simulink model "propeller_power_train"  (R2023b)
settings: Solver=ode1be  StartTime=0.0  StopTime=simlength  FixedStep=tc  MaxStep=tc
values from neighbouring files (symbols this model uses):
  angle_error = angle_error_deg/180*pi    (= 0.13962634016)    [init_2023_10_06.m]
  CTRPIFF_CLIP_RELEASE = 0.01    [init_2023_10_06.m]
  dead_time = dead_time_INV    (= 4.2e-07)    [init_2023_10_06.m]
  dead_time_INV = 0.42e-6    (= 4.2e-07)    [init_2023_10_06.m]
  DThs_init = 0    [init_2023_10_06.m]
  emf_fb_p = 0.2    [init_2023_10_06.m]
  emf_fb_p_ccaller_1 = 0.2    [init_2023_10_06.m]
  emf_fb_p_ccaller_2 = 0.4    [init_2023_10_06.m]
  emf_p = emf_fb_p*4/10    (= 0.08)    [init_2023_10_06.m]
  emf_p_ccaller_1 = emf_fb_p_ccaller_1*4/10    (= 0.08)    [init_2023_10_06.m]
  emf_p_ccaller_2 = emf_fb_p_ccaller_2*4/10    (= 0.16)    [init_2023_10_06.m]
  fPWM_INV = 30e3    (= 30000)    [init_2023_10_06.m]
  g0_reference_flt = fcut_reference_flt * ts_inv * 2*pi    (= 0.000837758040957)    [init_2023_10_06.m]
  g1_reference_flt = 1 - g0_reference_flt    (= 0.999162241959)    [init_2023_10_06.m]
  id_ref_if_pu = iload_rms_ref*sqrt(2)/ibez    [init_2023_10_06.m]
  kg = K(1)    [init_2023_10_06.m]
  ki_id = 35    [init_2023_10_06.m]
  ki_iq = 35    [init_2023_10_06.m]
  kp_id = 0.15    [init_2023_10_06.m]
  kp_iq = 0.15    [init_2023_10_06.m]
  kw = K(2)    [init_2023_10_06.m]
  motorc_m_scale = 2/3*Vdc_bez/ubez    [init_2023_10_06.m]
  number_of_cells = 92    [init_2023_10_06.m]
  omega_flt_fcut = 4    [init_2023_10_06.m]
  omega_flt_g0 = omega_flt_fcut * ts_inv * 2*pi    (= 0.000837758040957)    [init_2023_10_06.m]
  omega_flt_g1 = 1 - omega_flt_g0    (= 0.999162241959)    [init_2023_10_06.m]
  omega_ref_if_pu = 300*2*pi/omega_bez    [init_2023_10_06.m]
  phase_compensation_omega = 0    [init_2023_10_06.m]
  pwm_out_lim = 1    [init_2023_10_06.m]
  Q = 10    [init_2023_10_06.m]
  q1Kalman = ts_inv^2    (= 1.11111111111e-09)    [init_2023_10_06.m]
  q2Kalman = ts_inv^1    (= 3.33333333333e-05)    [init_2023_10_06.m]
  q3Kalman = 0    [init_2023_10_06.m]
  rKalman = 1    [init_2023_10_06.m]
  Tambient = 1    [init_2023_10_06.m]
  tc = ts_inv/400    (= 8.33333333333e-08)    [init_2023_10_06.m]
  time_init = 0.025    [init_2023_10_06.m]
  torque_ref = 64/ibez*1.1    [init_2023_10_06.m]
  ts_inv = 1/fPWM_INV    (= 3.33333333333e-05)    [init_2023_10_06.m]
  tsample = ts_inv    (= 3.33333333333e-05)    [init_2023_10_06.m]
  Vdc_bez = 400    [init_2023_10_06.m]
undefined symbols (not defined in the file or in its folder): b, b_square, ibez, Jm, Ld_norm, Lq_norm, Ls_norm, magnitude, omega_bez, phi_bez, phi_m, phi_m_norm, R_RLload, Rload_eq, Rs_norm, tau_bez, weigth
libraries: fl_lib x90, nesl_utility x80, ee_lib x11, pmsm_uvw_with_harmonics_lib x2, lithium_ion_cell_lib x1, simulink x1, flexshaft_lib x1
(part 3 of 5)

== system propeller_power_train/driver control/current_ctrl/sample_hold_normalization ==
  iu : Inport
  iv : Inport  Port=2
  iw : Inport  Port=3
  Gain : Gain  Gain=1/ibez
  Gain1 : Gain  Gain=1/ibez
  Gain2 : Gain  Gain=1/ibez
  Gain3 : Gain  Commented=through  Gain=-1
  Gain4 : Gain  Commented=through  Gain=-1
  Gain5 : Gain  Commented=through  Gain=-1
  Unit Delay{,1..5} (6 alike) : UnitDelay  SampleTime=ts_inv  HasFrameUpgradeWarning=on
  Zero-Order Hold : ZeroOrderHold  SampleTime=ts_inv
  Zero-Order Hold1 : ZeroOrderHold  SampleTime=ts_inv
  Zero-Order Hold2 : ZeroOrderHold  SampleTime=ts_inv
  iu_pu : Outport
  iv_pu : Outport  Port=2
  iw_pu : Outport  Port=3
  wires:
  iv/1 -> Zero-Order Hold1/1
  iw/1 -> Zero-Order Hold2/1
  Zero-Order Hold/1 -> Unit Delay/1
  Zero-Order Hold2/1 -> Unit Delay4/1
  Unit Delay/1 -> Unit Delay2/1
  Zero-Order Hold1/1 -> Unit Delay1/1
  Unit Delay1/1 -> Unit Delay3/1
  Unit Delay4/1 -> Unit Delay5/1
  iu/1 -> Zero-Order Hold/1
  Gain/1 -> Gain3/1
  Gain1/1 -> Gain4/1
  Gain2/1 -> Gain5/1
  Gain3/1 -> iu_pu/1
  Gain4/1 -> iv_pu/1
  Gain5/1 -> iw_pu/1
  Unit Delay2/1 -> Gain/1
  Unit Delay3/1 -> Gain1/1
  Unit Delay5/1 -> Gain2/1

== system propeller_power_train/driver control/current_ctrl/vector_current_ctrl ==
  iq_ref : Inport
  id_ref : Inport  Port=2
  MTPA : Subsystem
      settings: PortSchema="{\"entries\":[{\"content\":{\"sides\":[{\"content\":{\"connectorIds\":[\"In1\"]},\"type\":\"ConnectorPlacement.EquallySpacedRectSide\",\"uuid\":\"b7b50820-32cf-4b06-b710-c36db40508fb\"},{\"content\":{\"connectorIds\":[\"Out1\"],\"side\":\"RIGHT\"},\"type\":\"ConnectorPlacement.EquallySpacedRectSide\",\"uuid\":\"9680176d-6365-4ae4-8330-83815ae14f93\"},{\"content\":{\"connectorIds\":[\"In2\"],\"side\":\"TOP\"},\"type\":\"ConnectorPlacement.EquallySpacedRectSide\",\"uuid\":\"503d8594-1c43-4fac-b8a6-77f5afdeeec1\"}]},\"type\":\"ConnectorPlacement.EquallySpacedConnector\",\"uuid\":\"c97785bf-1f92-4066-ba86-64cef6027105\"}],\"packageUris\":[\"http://schema.mathworks.com/mf0/Connector/R2020b\"],\"version\":\"1.0\"}"
  Variant Source : VariantSource  ShowConditionOnBlock=on
  Variant Source1 : VariantSource  ShowConditionOnBlock=on
  dq_vector_pi : Subsystem
  dq_vector_pi_ccaller : Subsystem
  id_ref_pu/id_pu : Scope  NumInputPorts=2
  iq_ref_pu/iq_pu : Scope  NumInputPorts=2
  ud : Outport
  uq : Outport  Port=2
  tag scope: id_ref_inverter_pu=global, iq_ref_inverter_pu=global, ud_inverter_pu=global, uq_inverter_pu=global
  wires:
  [iq_inverter_pu] -> dq_vector_pi/3(iq), iq_ref_pu/iq_pu/2, dq_vector_pi_ccaller/3(iq)  "iq_inverter_pu"
  [id_inverter_pu] -> dq_vector_pi/1(id), dq_vector_pi_ccaller/1(id), id_ref_pu/id_pu/2  "id_inverter_pu"
  iq_ref/1 -> MTPA/1(iq_ref), dq_vector_pi/4(iq_ref), [iq_ref_inverter_pu], iq_ref_pu/iq_pu/1, dq_vector_pi_ccaller/4(iq_ref)  "iq_ref"
  MTPA/1(id_ref) -> dq_vector_pi/2(id_ref), dq_vector_pi_ccaller/2(id_ref), [id_ref_inverter_pu], id_ref_pu/id_pu/1  "id_ref"
  id_ref/1 -> MTPA/2(id_ref_ext)
  Variant Source/1 -> [ud_inverter_pu], ud/1
  dq_vector_pi_ccaller/1(ud_ctrl_out) -> Variant Source/1
  dq_vector_pi_ccaller/2(uq_ctrl_out) -> Variant Source1/1
  Variant Source1/1 -> [uq_inverter_pu], uq/1
  dq_vector_pi/1(ctrl_d_u) -> Variant Source/2
  dq_vector_pi/2(ctrl_q_u) -> Variant Source1/2

== system propeller_power_train/driver control/torque_reference_generator/reference_d_flt ==
  input : Inport
  Gain3 : Gain  Gain=g1_reference_flt
  Gain6 : Gain  Gain=g0_reference_flt
  Sum : Sum  Inputs=|++
  Unit Delay1 : UnitDelay  SampleTime=ts_inv  HasFrameUpgradeWarning=on
  output : Outport  VectorParamsAs1DForOutWhenUnconnected=off
  wires:
  Gain6/1 -> Sum/1
  input/1 -> Gain6/1
  Unit Delay1/1 -> Gain3/1
  Gain3/1 -> Sum/2
  Sum/1 -> Unit Delay1/1, output/1

== system propeller_power_train/driver control/torque_reference_generator/reference_q_flt ==
  input : Inport
  Gain3 : Gain  Gain=g1_reference_flt
  Gain6 : Gain  Gain=g0_reference_flt
  Sum : Sum  Inputs=|++
  Unit Delay1 : UnitDelay  SampleTime=ts_inv  HasFrameUpgradeWarning=on
  output : Outport  VectorParamsAs1DForOutWhenUnconnected=off
  wires:
  Sum/1 -> output/1, Unit Delay1/1
  Gain3/1 -> Sum/2
  Unit Delay1/1 -> Gain3/1
  input/1 -> Gain6/1
  Gain6/1 -> Sum/1

== system propeller_power_train/inverter/Gyro based inverter/gyro1 ==
  m : Inport
  Controlled Current Source : fl_lib/Electrical/Electrical Sources/Controlled Current Source
  Controlled Voltage Source : fl_lib/Electrical/Electrical Sources/Controlled Voltage Source
  Current Sensor : fl_lib/Electrical/Electrical Sensors/Current Sensor
  PS Product : fl_lib/Physical Signals/Functions/PS Product
  PS Product1 : fl_lib/Physical Signals/Functions/PS Product
  Simulink-PS Converter : nesl_utility/Simulink-PS Converter  PhysicalDomain=network_engine_domain  SubClassName=ps_input  LeftPortType=input  RightPortType=output  PseudoPeriodic=off  Frequencies=[]  NoiseDistribution=none  NoiseParameters=[]  Unit=1  AffineConversion=on  FilteringAndDerivatives=provide  SimscapeFilterOrder=1  InputFilterTimeConstant=0.001  UdotUserProvided=0
  Voltage Sensor : fl_lib/Electrical/Electrical Sensors/Voltage Sensor
  uin+ : PMIOPort  Side=Left
  uin- : PMIOPort  Port=2  Side=Left
  uout+ : PMIOPort  Port=3  Side=Right
  uout- : PMIOPort  Port=4  Side=Right
  wires:
  m/1 -> Simulink-PS Converter/1
  connections:
  Voltage Sensor/RConn2 -- Controlled Current Source/LConn1 -- uin-/RConn1
  Voltage Sensor/LConn1 -- Controlled Current Source/RConn2 -- uin+/RConn1
  Controlled Voltage Source/LConn1 -- Current Sensor/LConn1
  Controlled Voltage Source/RConn2 -- uout-/RConn1
  Current Sensor/RConn2 -- uout+/RConn1
  Simulink-PS Converter/RConn1 -- PS Product/LConn1 -- PS Product1/LConn2
  Voltage Sensor/RConn1 -- PS Product/LConn2
  PS Product1/RConn1 -- Controlled Current Source/RConn1
  PS Product/RConn1 -- Controlled Voltage Source/RConn1
  Current Sensor/RConn1 -- PS Product1/LConn1

== system propeller_power_train/inverter/Gyro based inverter/gyro2 ==
  m : Inport
  Controlled Current Source : fl_lib/Electrical/Electrical Sources/Controlled Current Source
  Controlled Voltage Source : fl_lib/Electrical/Electrical Sources/Controlled Voltage Source
  Current Sensor : fl_lib/Electrical/Electrical Sensors/Current Sensor
  PS Product : fl_lib/Physical Signals/Functions/PS Product
  PS Product1 : fl_lib/Physical Signals/Functions/PS Product
  Simulink-PS Converter : nesl_utility/Simulink-PS Converter  PhysicalDomain=network_engine_domain  SubClassName=ps_input  LeftPortType=input  RightPortType=output  PseudoPeriodic=off  Frequencies=[]  NoiseDistribution=none  NoiseParameters=[]  Unit=1  AffineConversion=on  FilteringAndDerivatives=provide  SimscapeFilterOrder=1  InputFilterTimeConstant=0.001  UdotUserProvided=0
  Voltage Sensor : fl_lib/Electrical/Electrical Sensors/Voltage Sensor
  uin+ : PMIOPort  Side=Left
  uin- : PMIOPort  Port=2  Side=Left
  uout+ : PMIOPort  Port=3  Side=Right
  uout- : PMIOPort  Port=4  Side=Right
  wires:
  m/1 -> Simulink-PS Converter/1
  connections:
  Current Sensor/RConn1 -- PS Product1/LConn1
  PS Product/RConn1 -- Controlled Voltage Source/RConn1
  PS Product1/RConn1 -- Controlled Current Source/RConn1
  Voltage Sensor/RConn1 -- PS Product/LConn2
  PS Product1/LConn2 -- PS Product/LConn1 -- Simulink-PS Converter/RConn1
  Current Sensor/RConn2 -- uout+/RConn1
  Controlled Voltage Source/RConn2 -- uout-/RConn1
  Controlled Voltage Source/LConn1 -- Current Sensor/LConn1
  uin+/RConn1 -- Controlled Current Source/RConn2 -- Voltage Sensor/LConn1
  uin-/RConn1 -- Controlled Current Source/LConn1 -- Voltage Sensor/RConn2

== system propeller_power_train/inverter/Gyro based inverter/gyro3 ==
  m : Inport
  Controlled Current Source : fl_lib/Electrical/Electrical Sources/Controlled Current Source
  Controlled Voltage Source : fl_lib/Electrical/Electrical Sources/Controlled Voltage Source
  Current Sensor : fl_lib/Electrical/Electrical Sensors/Current Sensor
  PS Product : fl_lib/Physical Signals/Functions/PS Product
  PS Product1 : fl_lib/Physical Signals/Functions/PS Product
  Simulink-PS Converter : nesl_utility/Simulink-PS Converter  PhysicalDomain=network_engine_domain  SubClassName=ps_input  LeftPortType=input  RightPortType=output  PseudoPeriodic=off  Frequencies=[]  NoiseDistribution=none  NoiseParameters=[]  Unit=1  AffineConversion=on  FilteringAndDerivatives=provide  SimscapeFilterOrder=1  InputFilterTimeConstant=0.001  UdotUserProvided=0
  Voltage Sensor : fl_lib/Electrical/Electrical Sensors/Voltage Sensor
  uin+ : PMIOPort  Side=Left
  uin- : PMIOPort  Port=2  Side=Left
  uout+ : PMIOPort  Port=3  Side=Right
  uout- : PMIOPort  Port=4  Side=Right
  wires:
  m/1 -> Simulink-PS Converter/1
  connections:
  Voltage Sensor/RConn2 -- Controlled Current Source/LConn1 -- uin-/RConn1
  Voltage Sensor/LConn1 -- Controlled Current Source/RConn2 -- uin+/RConn1
  Controlled Voltage Source/LConn1 -- Current Sensor/LConn1
  Controlled Voltage Source/RConn2 -- uout-/RConn1
  Current Sensor/RConn2 -- uout+/RConn1
  Simulink-PS Converter/RConn1 -- PS Product/LConn1 -- PS Product1/LConn2
  Voltage Sensor/RConn1 -- PS Product/LConn2
  PS Product1/RConn1 -- Controlled Current Source/RConn1
  PS Product/RConn1 -- Controlled Voltage Source/RConn1
  Current Sensor/RConn1 -- PS Product1/LConn1

== system propeller_power_train/inverter/MOS based inverter/inverter ==
  inverter_mosfet_leg_thermal : Subsystem
  inverter_without_mosfet_leg_thermal : Subsystem  Commented=on
  udc(+) : PMIOPort  Side=Left
  udc(-) : PMIOPort  Port=2  Side=Left
  u : PMIOPort  Port=3  Side=Right
  v : PMIOPort  Port=4  Side=Right
  w : PMIOPort  Port=5  Side=Right
  connections:
  udc(+)/RConn1 -- inverter_without_mosfet_leg_thermal/LConn1 -- inverter_mosfet_leg_thermal/LConn1
  inverter_mosfet_leg_thermal/RConn1 -- inverter_without_mosfet_leg_thermal/RConn1 -- u/RConn1
  inverter_mosfet_leg_thermal/RConn2 -- inverter_without_mosfet_leg_thermal/RConn2 -- v/RConn1
  w/RConn1 -- inverter_without_mosfet_leg_thermal/RConn3 -- inverter_mosfet_leg_thermal/RConn3
  udc(-)/RConn1 -- inverter_without_mosfet_leg_thermal/LConn2 -- inverter_mosfet_leg_thermal/LConn2

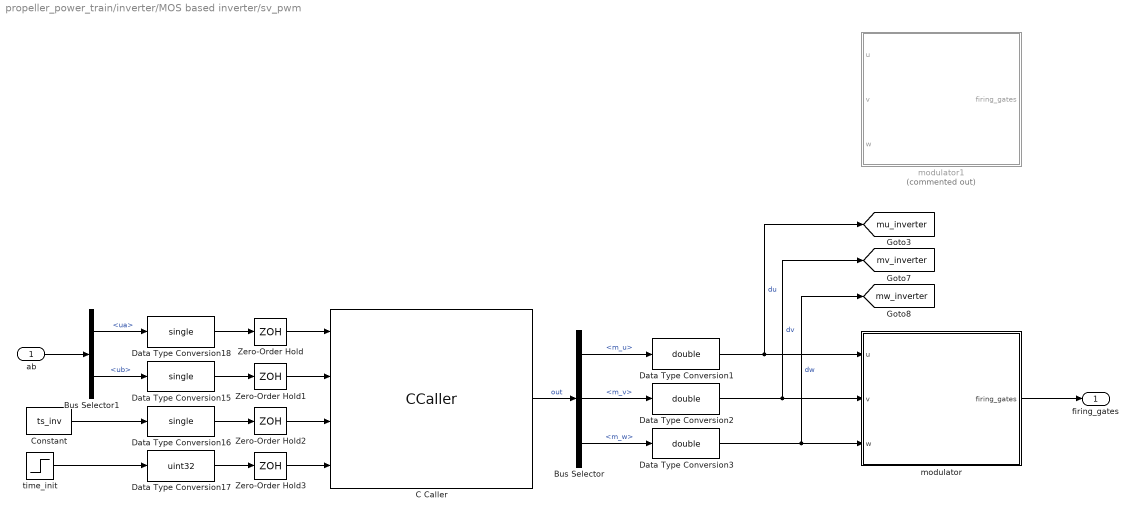
== system propeller_power_train/inverter/MOS based inverter/sv_pwm ==
  ab : Inport
  Bus Selector : BusSelector  OutputSignals=m_u,m_v,m_w
  Bus Selector1 : BusSelector  OutputSignals=ua,ub
  C Caller : CCaller  FunctionName=sv_pwm_process_simulink  PortSpecificationStruct="%)30     .    N @   8    (     @         %    \"     4    !     0         %  0 \"0    $    _    07)G3F%M90  4&]R=$YA;64 4V-O<&4     26YD97@     5'EP90      4VEZ90      27-';&]B86P   X    P    !@    @    $          4    (     0    ,    !         !   P!O=70 #@   #     &    \"     0         !0    @    !     P    $         $  # &]U=  .    .     8    (    !          %    \"     $    &     0         0   ...(+2630 chars)"  SampleTime=ts_inv
  Constant : Constant  Value=ts_inv
  Data Type Conversion1 : DataTypeConversion  OutDataTypeStr=double  SaturateOnIntegerOverflow=off  RndMeth=Floor
  Data Type Conversion15 : DataTypeConversion  OutDataTypeStr=single  SaturateOnIntegerOverflow=off  RndMeth=Floor
  Data Type Conversion16 : DataTypeConversion  OutDataTypeStr=single  SaturateOnIntegerOverflow=off  RndMeth=Floor
  Data Type Conversion17 : DataTypeConversion  OutDataTypeStr=uint32  SaturateOnIntegerOverflow=off  RndMeth=Floor
  Data Type Conversion18 : DataTypeConversion  OutDataTypeStr=single  SaturateOnIntegerOverflow=off  RndMeth=Floor
  Data Type Conversion2 : DataTypeConversion  OutDataTypeStr=double  SaturateOnIntegerOverflow=off  RndMeth=Floor
  Data Type Conversion3 : DataTypeConversion  OutDataTypeStr=double  SaturateOnIntegerOverflow=off  RndMeth=Floor
  Zero-Order Hold{,1..3} (4 alike) : ZeroOrderHold  SampleTime=ts_inv
  modulator : Subsystem
  modulator1 : Subsystem  Commented=on
  time_init : Step  Time=time_init  SampleTime=0
  firing_gates : Outport
  tag scope: mu_inverter=global, mv_inverter=global, mw_inverter=global
  wires:
  Data Type Conversion1/1 -> [mu_inverter], modulator/1(u)  "du"
  Zero-Order Hold/1 -> C Caller/1
  Zero-Order Hold2/1 -> C Caller/3
  Constant/1 -> Data Type Conversion16/1
  Bus Selector/1 -> Data Type Conversion1/1  "<m_u>"
  Data Type Conversion18/1 -> Zero-Order Hold/1
  Bus Selector/3 -> Data Type Conversion3/1  "<m_w>"
  Data Type Conversion2/1 -> [mv_inverter], modulator/2(v)  "dv"
  Data Type Conversion16/1 -> Zero-Order Hold2/1
  Zero-Order Hold1/1 -> C Caller/2
  Data Type Conversion17/1 -> Zero-Order Hold3/1
  Zero-Order Hold3/1 -> C Caller/4
  Data Type Conversion15/1 -> Zero-Order Hold1/1
  C Caller/1 -> Bus Selector/1  "out"
  Bus Selector/2 -> Data Type Conversion2/1  "<m_v>"
  Data Type Conversion3/1 -> [mw_inverter], modulator/3(w)  "dw"
  modulator/1(firing_gates) -> firing_gates/1
  ab/1 -> Bus Selector1/1
  Bus Selector1/1 -> Data Type Conversion18/1  "<ua>"
  Bus Selector1/2 -> Data Type Conversion15/1  "<ub>"
  time_init/1 -> Data Type Conversion17/1

== system propeller_power_train/inverter/MOS based inverter/threePhsModulator ==
  uab_pu : Inport
  Bus Creator1 : BusCreator  Inputs=2
  Bus Creator2 : BusCreator  Inputs=2
  Bus Creator3 : BusCreator  Inputs=3
  Bus Creator4 : BusCreator  Inputs=2
  Demux1 : Demux  Outputs=2
  Gain6 : Gain  Gain=1/sqrt(3)*2
  Gain7 : Gain  Gain=1/sqrt(3)*2
  Gain8 : Gain  Gain=1/sqrt(3)*2
  PWM generator 1 : Subsystem  mask{f=fPWM_INV, ph=0, m_up=1, m_low=-1, dead_time=dead_time, gate_voltage=15}
      mask prompts: f "Frequency"; ph "Phase"; m_up "Max Input Modulation Value"; m_low "Min Input Modulation Value"; dead_time "Dead Time"; gate_voltage "Gate Voltage"
  PWM generator 2 : Subsystem  mask{f=fPWM_INV, ph=0, m_up=1, m_low=-1, dead_time=dead_time, gate_voltage=15}
      mask prompts: f "Frequency"; ph "Phase"; m_up "Max Input Modulation Value"; m_low "Min Input Modulation Value"; dead_time "Dead Time"; gate_voltage "Gate Voltage"
  PWM generator 3 : Subsystem  mask{f=fPWM_INV, ph=0, m_up=1, m_low=-1, dead_time=dead_time, gate_voltage=15}
      mask prompts: f "Frequency"; ph "Phase"; m_up "Max Input Modulation Value"; m_low "Min Input Modulation Value"; dead_time "Dead Time"; gate_voltage "Gate Voltage"
  Sum : Sum  Inputs=|+-
  Sum1 : Sum  Inputs=|+-
  Sum2 : Sum  Inputs=|+-
  Third harmonic injecting : Subsystem
  du/dv/dw : Scope  NumInputPorts=3
  uvw2alphabeta1 : MATLAB Function  TreatAsAtomicUnit=on  SystemSampleTime=ts_inv
  mout : Outport
  wires:
  uab_pu/1 -> Demux1/1
  Demux1/1 -> uvw2alphabeta1/1(alpha)
  Demux1/2 -> uvw2alphabeta1/2(beta)
  Third harmonic injecting/1(thind_H) -> Sum1/2, Sum/2, Sum2/2
  uvw2alphabeta1/1(u) -> Third harmonic injecting/1(m1), Sum/1  "ur"
  uvw2alphabeta1/2(v) -> Third harmonic injecting/2(m2), Sum1/1  "vr"
  uvw2alphabeta1/3(w) -> Sum2/1, Third harmonic injecting/3(m3)  "wr"
  Sum/1 -> Gain6/1
  Bus Creator3/1 -> mout/1
  PWM generator 1/1(m1) -> Bus Creator1/1  "gate_command_1"
  PWM generator 1/2(m2) -> Bus Creator1/2  "gate_command_2"
  Bus Creator1/1 -> Bus Creator3/1  "legA"
  PWM generator 2/2(m2) -> Bus Creator2/2  "gate_command_4"
  PWM generator 2/1(m1) -> Bus Creator2/1  "gate_command_3"
  PWM generator 3/1(m1) -> Bus Creator4/1  "gate_command_5"
  PWM generator 3/2(m2) -> Bus Creator4/2  "gate_command_6"
  Bus Creator2/1 -> Bus Creator3/2  "legB"
  Bus Creator4/1 -> Bus Creator3/3  "legC"
  Sum1/1 -> Gain7/1
  Sum2/1 -> Gain8/1
  Gain6/1 -> du/dv/dw/1, PWM generator 1/1(m_index)  "mu"
  Gain8/1 -> du/dv/dw/3, PWM generator 3/1(m_index)  "mw"
  Gain7/1 -> PWM generator 2/1(m_index), du/dv/dw/2  "mv"

== system propeller_power_train/battery_system/battery_system/LithiumIonBattery/SOC_estimator ==
  Kalman_observer : Subsystem
  SOC*/SOC : Scope  Commented=on  NumInputPorts=2
  Selector1 : Selector  InputPortWidth=3  IndexOptions=Index vector (dialog)  Indices=3  OutputSizes=1
  h_hat/h : Scope  Commented=on  NumInputPorts=2
  i_out/v_out : Scope  Commented=on  NumInputPorts=2
  soc/iout : Scope  Commented=on  NumInputPorts=2
  wires:
  Kalman_observer/2(SOC) -> SOC*/SOC/2
  Kalman_observer/1(x(k+1|k)) -> Selector1/1
  [im] -> i_out/v_out/1  "im+noise"
  [h] -> h_hat/h/2
  [SOC] -> soc/iout/1, SOC*/SOC/1
  Selector1/1 -> h_hat/h/1  "h_hat(z)"
  [vout] -> Kalman_observer/1(vout(k)), i_out/v_out/2
  [icell] -> soc/iout/2

== system propeller_power_train/battery_system/battery_system/LithiumIonBattery/lithium ion cell analytical ocv ==
  Current Sensor : fl_lib/Electrical/Electrical Sensors/Current Sensor
  Electrical Reference : fl_lib/Electrical/Electrical Elements/Electrical Reference
  PS Constant : fl_lib/Physical Signals/Sources/PS Constant  constant=298.15 K
  PS-Simulink Converter{,1..4} (5 alike) : nesl_utility/PS-Simulink Converter  PhysicalDomain=network_engine_domain  SubClassName=ps_output  LeftPortType=input  RightPortType=output  PseudoPeriodic=off  Frequencies=[]  VectorFormat=1-D array  Unit=inherit  AffineConversion=off
  Voltage Sensor : fl_lib/Electrical/Electrical Sensors/Voltage Sensor
  lithium-ion battery with analytical OCV : lithium_ion_cell_lib/lithium-ion Cell with analytical OCV  Qcell=Q hr*A  N=number_of_cells  E_1=E1 V  E0=E0 V  E1=E1 V  E2=E2 V  E3=E3 V  Elog=Elog V  R0=R0 Ohm  R1=R1 Ohm  C1=C1 F  M=M V  alpha=alpha  u_specify=off  u_priority=High  u=Vdc V  u_nominal_specify=off  u_nominal_unit=V  u_nominal_value=1  u_ocv_specify=off  u_ocv_priority=High  u_ocv=Vdc V  u_ocv_nominal_specify=off  u_ocv_nominal_unit=V  u_ocv_nominal_value=1  icell_specify=off  icell_priority=None  icell=0 A  icell_nominal_specify=off  icell_nominal_unit=A  icell_nominal_value=1  i_r1_specify=off  i_r1_priority=None  i_r1=0 A  i_r1_nominal_specify=off  i_r1_nominal_unit=A  i_r1_nominal_value=1  z_specify=on  z_priority=High  z=soc_init  z_nominal_specify=off  z_nominal_unit=1  z_nominal_value=1  h_specify=off  h_priority=High  h=0  h_nominal_specify=off  h_nominal_unit=1  h_nominal_value=1
      settings: InternalSimscapePortConfiguration="{\"Bottom\":[],\"Left\":[{\"id\":\"T\",\"label\":\"T\",\"type\":\"input\"}],\"Right\":[{\"id\":\"u_p\",\"label\":\"u+\",\"type\":\"foundation.electrical.electrical\"},{\"id\":\"u_n\",\"label\":\"u-\",\"type\":\"foundation.electrical.electrical\"},{\"id\":\"z_out\",\"label\":\"SOC\",\"type\":\"output\"},{\"id\":\"i_r1_out\",\"label\":\"i_r1\",\"type\":\"output\"},{\"id\":\"h_out\",\"label\":\"hysteresis\",\"type\":\"output\"}],\"Top\":[]}"
  white_noise : Subsystem
  U+ : PMIOPort  Side=Right
  U- : PMIOPort  Port=2  Side=Right
  tag scope: SOC=global, h=global, icell=global, im=global, vout=global
  wires:
  PS-Simulink Converter/1 -> [vout]  "vout(k)"
  PS-Simulink Converter1/1 -> white_noise/1(in)  "i(k)"
  white_noise/1(out) -> [im]
  PS-Simulink Converter4/1 -> [h]  "h(t)"
  PS-Simulink Converter2/1 -> [icell]  "icell"
  PS-Simulink Converter3/1 -> [SOC]  "SOC*"
  connections:
  lithium-ion battery with analytical OCV/LConn1 -- PS Constant/RConn1
  PS-Simulink Converter/LConn1 -- Voltage Sensor/RConn1
  Current Sensor/RConn2 -- Voltage Sensor/LConn1 -- U+/RConn1
  Electrical Reference/LConn1 -- Voltage Sensor/RConn2 -- U-/RConn1 -- lithium-ion battery with analytical OCV/RConn2
  Current Sensor/RConn1 -- PS-Simulink Converter1/LConn1
  lithium-ion battery with analytical OCV/RConn1 -- Current Sensor/LConn1
  lithium-ion battery with analytical OCV/RConn3 -- PS-Simulink Converter3/LConn1
  lithium-ion battery with analytical OCV/RConn4 -- PS-Simulink Converter2/LConn1
  lithium-ion battery with analytical OCV/RConn5 -- PS-Simulink Converter4/LConn1

== system propeller_power_train/driver control/bemf_observer/bemf_observer/double_integrator_observer ==
  theta : Inport
  Gain : Gain  Gain=kw
  Gain1 : Gain  Gain=kg
  Gain2 : Gain  Gain=omega_bez
  Gain3 : Gain  Gain=1/omega_bez
  Gain5 : Gain  Gain=ts_inv
  Sum : Sum  Inputs=-+|
  Sum1 : Sum  Inputs=|++
  Sum2 : Sum  Inputs=|++
  Sum8 : Sum  Inputs=++|
  Unit Delay1 : UnitDelay  SampleTime=ts_inv  HasFrameUpgradeWarning=on
  Unit Delay2 : UnitDelay  SampleTime=ts_inv  HasFrameUpgradeWarning=on
  bounder1 : MATLAB Function  TreatAsAtomicUnit=on  SystemSampleTime=ts_inv
  bounder2 : MATLAB Function  TreatAsAtomicUnit=on  SystemSampleTime=ts_inv
  omega_pu_hat : Outport  VectorParamsAs1DForOutWhenUnconnected=off
  theta_hat : Outport  Port=2  VectorParamsAs1DForOutWhenUnconnected=off
  wires:
  Gain1/1 -> Sum2/1
  theta/1 -> Sum/2  "theta_bemf"
  Sum8/1 -> bounder2/1(u)
  Sum1/1 -> Unit Delay2/1
  Gain/1 -> Gain3/1
  Unit Delay2/1 -> omega_pu_hat/1, Sum1/2, Gain5/1
  Sum2/1 -> Sum8/2
  bounder2/1(y) -> Unit Delay1/1
  bounder1/1(y) -> Gain/1, Gain1/1
  Gain2/1 -> Sum8/1
  Gain3/1 -> Sum1/1
  Gain5/1 -> Gain2/1
  Sum/1 -> bounder1/1(u)
  Unit Delay1/1 -> Sum2/2, theta_hat/1, Sum/1  "theta_hat"

== system propeller_power_train/driver control/bemf_observer/bemf_observer/omega_hat_flt ==
  omega_hat : Inport
  Gain3 : Gain  Gain=omega_flt_g1
  Gain6 : Gain  Gain=omega_flt_g0
  Sum : Sum  Inputs=|++
  Unit Delay1 : UnitDelay  SampleTime=ts_inv  HasFrameUpgradeWarning=on
  omega_hat_flt : Outport  VectorParamsAs1DForOutWhenUnconnected=off
  wires:
  Gain6/1 -> Sum/1
  omega_hat/1 -> Gain6/1
  Unit Delay1/1 -> Gain3/1
  Gain3/1 -> Sum/2
  Sum/1 -> Unit Delay1/1, omega_hat_flt/1

== system propeller_power_train/driver control/bemf_observer/bemf_observer/psi_alpha_hat ==
  ualpha : Inport
  ialpha : Inport  Port=2
  Gain1 : Gain  Gain=Rs_norm
  Gain2 : Gain  Gain=emf_fb_p
  Gain3 : Gain  Gain=emf_p
  Gain4 : Gain  Gain=omega_bez
  Gain5 : Gain  Gain=Ls_norm
  Gain6 : Gain  Gain=motorc_m_scale
  Gain7 : Gain  Gain=ts_inv
  Product : Product  RndMeth=Zero
  Sum : Sum  Inputs=|+-
  Sum1 : Sum  Inputs=|+-
  Sum2 : Sum  Inputs=++-  SaturateOnIntegerOverflow=on
  Sum3 : Sum  Inputs=|++
  Sum4 : Sum  Inputs=+-  SaturateOnIntegerOverflow=on
  Unit Delay1 : UnitDelay  SampleTime=ts_inv  HasFrameUpgradeWarning=on
  Unit Delay2 : UnitDelay  SampleTime=ts_inv  HasFrameUpgradeWarning=on
  Unit Delay3 : UnitDelay  SampleTime=ts_inv  HasFrameUpgradeWarning=on
  psi_s_alpha_hat : Outport  VectorParamsAs1DForOutWhenUnconnected=off
  psi_r_alpha_hat : Outport  Port=2  VectorParamsAs1DForOutWhenUnconnected=off
  wires:
  [psi_r_m_alpha] -> Sum1/1
  [psi_r_alpha_hat] -> Sum1/2
  Gain4/1 -> Gain7/1
  Sum2/1 -> Gain4/1
  Gain3/1 -> Sum2/3
  ialpha/1 -> Gain5/1, Gain1/1
  Gain1/1 -> Sum/2
  Sum/1 -> Sum2/2
  ualpha/1 -> Product/1
  Unit Delay1/1 -> Sum4/1, psi_s_alpha_hat/1, Gain3/1, Sum3/2
  Sum3/1 -> Unit Delay1/1  "psi_s_alpha_hat_hat"
  Sum1/1 -> Gain2/1
  Gain2/1 -> Sum2/1
  [vdc_pu] -> Product/2
  Gain7/1 -> Sum3/1
  Product/1 -> Gain6/1
  Gain6/1 -> Sum/1
  Gain5/1 -> Unit Delay2/1
  Sum4/1 -> Unit Delay3/1
  Unit Delay2/1 -> Sum4/2
  Unit Delay3/1 -> psi_r_alpha_hat/1

== system propeller_power_train/driver control/bemf_observer/bemf_observer/psi_beta_hat ==
  ubeta : Inport
  ibeta : Inport  Port=2
  Gain1 : Gain  Gain=Rs_norm
  Gain2 : Gain  Gain=emf_fb_p
  Gain3 : Gain  Gain=emf_p
  Gain4 : Gain  Gain=omega_bez
  Gain5 : Gain  Gain=Ls_norm
  Gain6 : Gain  Gain=motorc_m_scale
  Gain7 : Gain  Gain=ts_inv
  Product : Product  RndMeth=Zero
  Sum : Sum  Inputs=|+-
  Sum1 : Sum  Inputs=|+-
  Sum2 : Sum  Inputs=++-  SaturateOnIntegerOverflow=on
  Sum3 : Sum  Inputs=|++
  Sum4 : Sum  Inputs=+-  SaturateOnIntegerOverflow=on
  Unit Delay1 : UnitDelay  SampleTime=ts_inv  HasFrameUpgradeWarning=on
  Unit Delay2 : UnitDelay  SampleTime=ts_inv  HasFrameUpgradeWarning=on
  Unit Delay3 : UnitDelay  SampleTime=ts_inv  HasFrameUpgradeWarning=on
  psi_s_beta_hat : Outport  VectorParamsAs1DForOutWhenUnconnected=off
  psi_r_beta_hat : Outport  Port=2  VectorParamsAs1DForOutWhenUnconnected=off
  wires:
  Sum/1 -> Sum2/2
  Gain1/1 -> Sum/2
  ibeta/1 -> Gain5/1, Gain1/1
  Gain3/1 -> Sum2/3
  Sum2/1 -> Gain4/1
  Gain4/1 -> Gain7/1
  Sum1/1 -> Gain2/1
  [psi_r_beta_hat] -> Sum1/2
  [psi_r_m_beta] -> Sum1/1
  Unit Delay1/1 -> Gain3/1, Sum4/1, psi_s_beta_hat/1, Sum3/2
  Sum3/1 -> Unit Delay1/1
  Gain2/1 -> Sum2/1
  ubeta/1 -> Product/1
  [vdc_pu] -> Product/2
  Gain7/1 -> Sum3/1
  Product/1 -> Gain6/1
  Gain6/1 -> Sum/1
  Gain5/1 -> Unit Delay2/1
  Sum4/1 -> Unit Delay3/1
  Unit Delay2/1 -> Sum4/2
  Unit Delay3/1 -> psi_r_beta_hat/1

== system propeller_power_train/driver control/bemf_observer/bemf_observer/theta_bemf_hat ==
  psi_r_alpha_hat : Inport
  psi_r_beta_hat : Inport  Port=2
  omega_pu_hat : Inport  Port=3
  Sum : Sum  Inputs=|++
  Trigonometric Function : Trigonometry  Operator=atan2  OutputSignalType=real
  phase_compensation_omega : Gain  Gain=phase_compensation_omega
  theta_emf_hat : Outport  VectorParamsAs1DForOutWhenUnconnected=off
  wires:
  psi_r_alpha_hat/1 -> Trigonometric Function/2
  psi_r_beta_hat/1 -> Trigonometric Function/1
  Trigonometric Function/1 -> Sum/1
  omega_pu_hat/1 -> phase_compensation_omega/1
  phase_compensation_omega/1 -> Sum/2
  Sum/1 -> theta_emf_hat/1

== system propeller_power_train/driver control/bemf_observer/bemf_observer_Ccaller/Reset Trigger ==
  Step : Step  Time=time_init  Before=1  After=0  SampleTime=0
  Out1 : Outport
  wires:
  Step/1 -> Out1/1  "Reset"

== system propeller_power_train/driver control/current_ctrl/vector_current_ctrl/MTPA ==
  iq_ref : Inport
  id_ref_ext : Inport  Port=2
  Constant : Constant  Value=phi_m_norm
  Gain1 : Gain  Gain=1/(Ld_norm - Lq_norm)/2
  Gain2 : Gain  Gain=1/(Ld_norm - Lq_norm)/2
  Gain3 : Gain  Gain=0
  Math Function1 : Math  Operator=magnitude^2  SignedPower=on
  Math Function4 : Math  Operator=magnitude^2  SignedPower=on
  Sqrt : Sqrt
  Sum : Sum  Inputs=|++
  Sum1 : Sum  Inputs=|--
  Sum3 : Sum  Inputs=|++
  id_ref_pu < x < 0 : Saturate  UpperLimit=0  LowerLimit=-0.15
  id_ref : Outport  VectorParamsAs1DForOutWhenUnconnected=off
  wires:
  Sum1/1 -> id_ref_pu < x < 0/1
  id_ref_pu < x < 0/1 -> Gain3/1
  Math Function4/1 -> Sum/1
  Math Function1/1 -> Sum/2
  Gain1/1 -> Math Function4/1
  Sum/1 -> Sqrt/1
  Sqrt/1 -> Sum1/2
  iq_ref/1 -> Math Function1/1
  Gain2/1 -> Sum1/1
  Constant/1 -> Gain1/1, Gain2/1
  Gain3/1 -> Sum3/1
  Sum3/1 -> id_ref/1
  id_ref_ext/1 -> Sum3/2

== system propeller_power_train/driver control/current_ctrl/vector_current_ctrl/dq_vector_pi ==
  id : Inport
  id_ref : Inport  Port=2
  iq : Inport  Port=3
  iq_ref : Inport  Port=4
  Sum1 : Sum  Inputs=|+-
  Sum2 : Sum  Inputs=|+-
  bounder1 : Subsystem
  bounder2 : Subsystem
  pi_d : Subsystem
  pi_q : Subsystem
  switch : Subsystem
  vector lenght : Subsystem
  ctrl_d_u : Outport
  ctrl_q_u : Outport  Port=2
  wires:
  bounder2/2(clip) -> switch/2(clip 2)
  bounder2/1(mq_sat) -> ctrl_q_u/1
  pi_q/1(Vqs_out) -> bounder2/3(mq), vector lenght/2(mq)
  vector lenght/1(m_1) -> bounder1/2(m_1), bounder2/2(m_1)
  vector lenght/2(m) -> bounder1/3(m), bounder2/1(m)
  pi_d/1(ud_out) -> vector lenght/1(md), bounder1/1(md)
  switch/1(clip) -> pi_q/2(clip), pi_d/2(clip)
  bounder1/2(clip) -> switch/1(clip 1)
  Sum2/1 -> pi_q/1(iq_tilde)
  Sum1/1 -> pi_d/1(id_tilde)
  bounder1/1(md_sat) -> ctrl_d_u/1
  id_ref/1 -> Sum1/1
  id/1 -> Sum1/2
  iq_ref/1 -> Sum2/1
  iq/1 -> Sum2/2

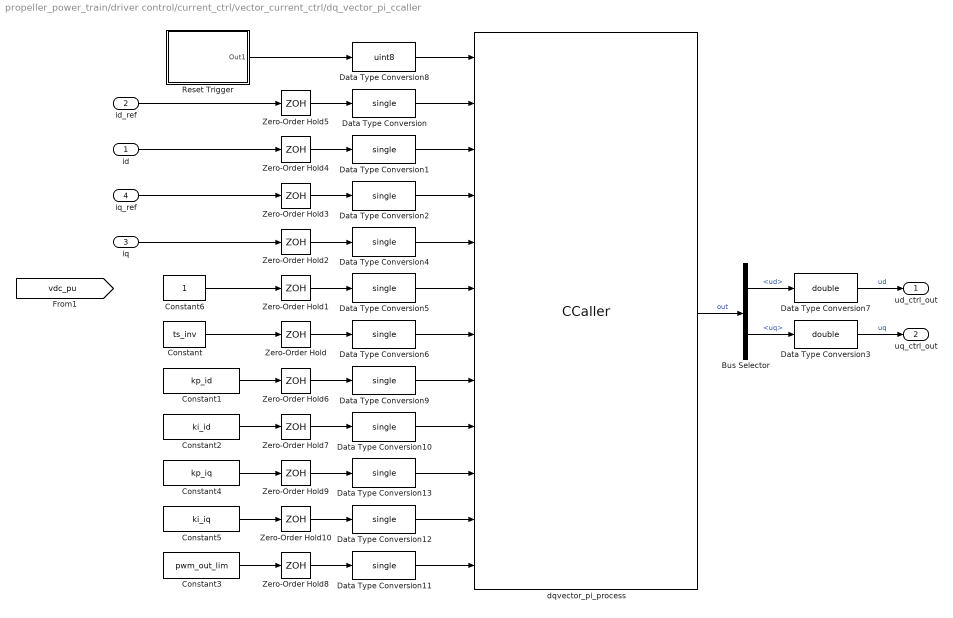
== system propeller_power_train/driver control/current_ctrl/vector_current_ctrl/dq_vector_pi_ccaller ==
  id : Inport
  id_ref : Inport  Port=2
  iq : Inport  Port=3
  iq_ref : Inport  Port=4
  Bus Selector : BusSelector  OutputSignals=ud,uq
  Constant : Constant  Value=ts_inv
  Constant1 : Constant  Value=kp_id
  Constant2 : Constant  Value=ki_id
  Constant3 : Constant  Value=pwm_out_lim
  Constant4 : Constant  Value=kp_iq
  Constant5 : Constant  Value=ki_iq
  Constant6 : Constant
  Data Type Conversion{,1..2,4..6,9..13} (11 alike) : DataTypeConversion  OutDataTypeStr=single  SaturateOnIntegerOverflow=off  RndMeth=Floor
  Data Type Conversion3 : DataTypeConversion  OutDataTypeStr=double  SaturateOnIntegerOverflow=off  RndMeth=Floor
  Data Type Conversion7 : DataTypeConversion  OutDataTypeStr=double  SaturateOnIntegerOverflow=off  RndMeth=Floor
  Data Type Conversion8 : DataTypeConversion  OutDataTypeStr=uint8  SaturateOnIntegerOverflow=off  RndMeth=Floor
  Reset Trigger : Subsystem
  Zero-Order Hold{,1..10} (11 alike) : ZeroOrderHold  SampleTime=ts_inv
  dqvector_pi_process : CCaller  FunctionName=dqvector_pi_process_simulink  PortSpecificationStruct="%)30     .    ,!8   8    (     @         %    \"     T    !     0         %  0 \"0    $    _    07)G3F%M90  4&]R=$YA;64 4V-O<&4     26YD97@     5'EP90      4VEZ90      27-';&]B86P   X    P    !@    @    $          4    (     0    ,    !         !   P!O=70 #@   #     &    \"     0         !0    @    !     P    $         $  # &]U=  .    .     8    (    !          %    \"     $    &     0         0   ...(+7280 chars)"  SampleTime=ts_inv
  ud_ctrl_out : Outport
  uq_ctrl_out : Outport  Port=2
  wires:
  Data Type Conversion5/1 -> dqvector_pi_process/6
  Data Type Conversion/1 -> dqvector_pi_process/2
  dqvector_pi_process/1 -> Bus Selector/1  "out"
  Data Type Conversion1/1 -> dqvector_pi_process/3
  Data Type Conversion4/1 -> dqvector_pi_process/5
  Data Type Conversion2/1 -> dqvector_pi_process/4
  Data Type Conversion6/1 -> dqvector_pi_process/7
  Zero-Order Hold/1 -> Data Type Conversion6/1
  Zero-Order Hold5/1 -> Data Type Conversion/1
  Zero-Order Hold4/1 -> Data Type Conversion1/1
  Zero-Order Hold3/1 -> Data Type Conversion2/1
  Zero-Order Hold2/1 -> Data Type Conversion4/1
  Zero-Order Hold1/1 -> Data Type Conversion5/1
  Constant6/1 -> Zero-Order Hold1/1
  Constant/1 -> Zero-Order Hold/1
  id_ref/1 -> Zero-Order Hold5/1
  iq_ref/1 -> Zero-Order Hold3/1
  id/1 -> Zero-Order Hold4/1
  iq/1 -> Zero-Order Hold2/1
  Bus Selector/2 -> Data Type Conversion3/1  "<uq>"
  Bus Selector/1 -> Data Type Conversion7/1  "<ud>"
  Data Type Conversion7/1 -> ud_ctrl_out/1  "ud"
  Data Type Conversion3/1 -> uq_ctrl_out/1  "uq"
  Reset Trigger/1(Out1) -> Data Type Conversion8/1
  Data Type Conversion8/1 -> dqvector_pi_process/1
  Constant1/1 -> Zero-Order Hold6/1
  Zero-Order Hold6/1 -> Data Type Conversion9/1
  Data Type Conversion9/1 -> dqvector_pi_process/8
  Data Type Conversion10/1 -> dqvector_pi_process/9
  Zero-Order Hold7/1 -> Data Type Conversion10/1
  Zero-Order Hold8/1 -> Data Type Conversion11/1
  Constant2/1 -> Zero-Order Hold7/1
  Constant3/1 -> Zero-Order Hold8/1
  Data Type Conversion11/1 -> dqvector_pi_process/12
  Constant5/1 -> Zero-Order Hold10/1
  Zero-Order Hold10/1 -> Data Type Conversion12/1
  Zero-Order Hold9/1 -> Data Type Conversion13/1
  Constant4/1 -> Zero-Order Hold9/1
  Data Type Conversion13/1 -> dqvector_pi_process/10
  Data Type Conversion12/1 -> dqvector_pi_process/11
